simulink model "modeloexp10"  (R2015a)
settings: Solver=ode1  SolverMode=SingleTasking  StartTime=0.0  StopTime=10  FixedStep=0.01  RelTol=1e-3
values from neighbouring files (symbols this model uses):
  alfa = 0.2818    [exp10.m]
  K = 54.96    [exp10.m]
  Kc = 3    [exp10.m]
  KNL = 59.7881    [exp10.m]
  Kp = 1.604    [exp10.m]
  T = 0.27    [exp10.m]
  To = 0.134    [exp10.m]
  U = 1.59    [exp10.m]
undefined symbols (not defined in the file): phi
libraries: simulink x1
settings Model: CovExternalEMLEnable=on  Creator=rpm  LastModifiedBy=sasuk
settings DataIOCC: LimitDataPoints=off  SignalLoggingSaveFormat=ModelDataLogs  SaveOutput=off  SignalLogging=off  DSMLogging=off  SaveTime=off  TimeSaveName=t
settings OptimizationCC: ExpressionDepthLimit=2147483647  InitFltsAndDblsToZero=on
settings DebuggingCC: UnderspecifiedInitializationDetection=Classic  MergeDetectMultiDrivingBlocksExec=none  FcnCallInpInsideContextMsg=EnableAllAsWarning  StateNameClashWarn=warning
settings GRTTargetCC: CombineOutputUpdateFcns=off  GRTInterface=on

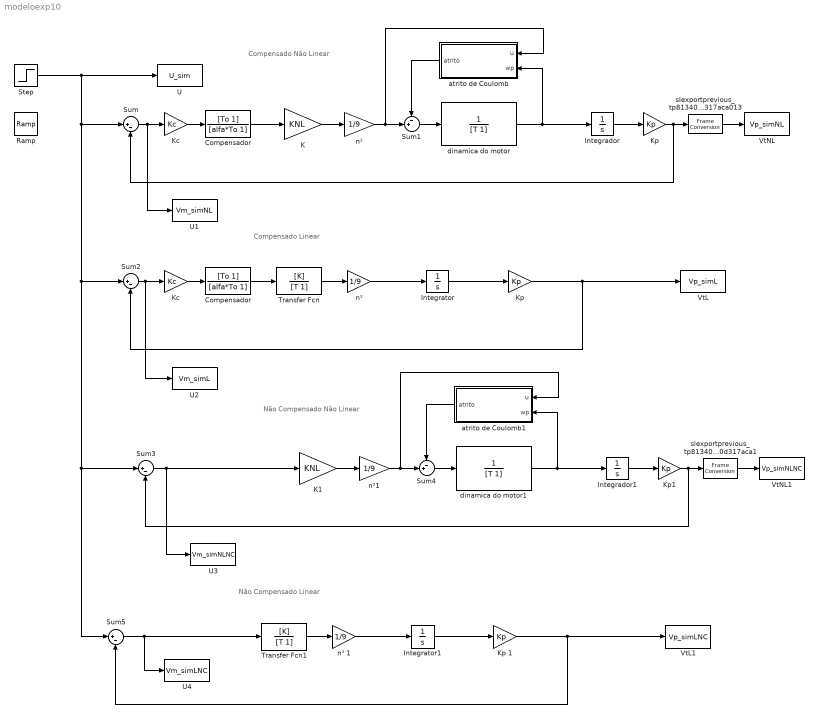
== system modeloexp10 ==
  note: Não Compensado
      | Não Linear
  note: Compensado Linear
  note: Compensado
      | Não
      | Linear
  note: Não Compensado Linear
  Compensador : TransferFcn  Numerator=[To 1]  Denominator=[alfa*To 1]
  "Compensador " : TransferFcn  Numerator=[To 1]  Denominator=[alfa*To 1]
  Integrador : Integrator
  Integrador1 : Integrator
  Integrator : Integrator
  Integrator1 : Integrator
  K : Gain  Gain=KNL
  K1 : Gain  Gain=KNL
  Kc : Gain  Gain=Kc
  "Kc " : Gain  Gain=Kc
  Kp : Gain  Gain=Kp
  "Kp " : Gain  Gain=Kp
  Kp 1 : Gain  Gain=Kp
  Kp1 : Gain  Gain=Kp
  Ramp : simulink/Sources/Ramp  slope=1  start=0  X0=0
  Step : Step  After=U  SampleTime=0
  Sum{,2..3,5} (4 alike) : Sum  Inputs=|+-
  Sum1 : Sum  Inputs=-+|
  Sum4 : Sum  Inputs=-+|
  Transfer Fcn : TransferFcn  Numerator=[K]  Denominator=[T 1]
  Transfer Fcn1 : TransferFcn  Numerator=[K]  Denominator=[T 1]
  U : ToWorkspace  VariableName=U_sim  SaveFormat=Timeseries  SampleTime=-1
  U1 : ToWorkspace  VariableName=Vm_simNL  SaveFormat=Timeseries  SampleTime=-1
  U2 : ToWorkspace  VariableName=Vm_simL  SaveFormat=Timeseries  SampleTime=-1
  U3 : ToWorkspace  VariableName=Vm_simNLNC  SaveFormat=Timeseries  SampleTime=-1
  U4 : ToWorkspace  VariableName=Vm_simLNC  SaveFormat=Timeseries  SampleTime=-1
  VtL : ToWorkspace  VariableName=Vp_simL  SaveFormat=Timeseries  SampleTime=-1
  VtL1 : ToWorkspace  VariableName=Vp_simLNC  SaveFormat=Timeseries  SampleTime=-1
  VtNL : ToWorkspace  VariableName=Vp_simNL  SaveFormat=Timeseries  SampleTime=-1
  VtNL1 : ToWorkspace  VariableName=Vp_simNLNC  SaveFormat=Timeseries  SampleTime=-1
  atrito de Coulomb : Subsystem  mask{phi=phi}
      mask Display: fprintf('phi = %3.1f', phi)
  atrito de Coulomb1 : Subsystem  mask{phi=phi}
      mask Display: fprintf('phi = %3.1f', phi)
  dinamica do motor : TransferFcn  Denominator=[T 1]
  dinamica do motor1 : TransferFcn  Denominator=[T 1]
  n² : Gain  Gain=1/9
  "n² " : Gain  Gain=1/9
  n² 1 : Gain  Gain=1/9
  n²1 : Gain  Gain=1/9
  slexportprevious_tp8134031d_9c58_445d_bef1_a0d317aca013 : FrameConversion  OutFrame=Sample-based
  slexportprevious_tp8134031d_9c58_445d_bef1_a0d317aca1 : FrameConversion  OutFrame=Sample-based
  wires:
  dinamica do motor/1 -> Integrador/1, atrito de Coulomb/2(wp)
  Integrador/1 -> Kp/1
  K/1 -> n²/1
  n²/1 -> atrito de Coulomb/1(u), Sum1/2
  atrito de Coulomb/1(atrito) -> Sum1/1
  Sum1/1 -> dinamica do motor/1
  Kp/1 -> Sum/2, slexportprevious_tp8134031d_9c58_445d_bef1_a0d317aca013/1
  slexportprevious_tp8134031d_9c58_445d_bef1_a0d317aca013/1 -> VtNL/1
  Transfer Fcn/1 -> "n² "/1
  "n² "/1 -> Integrator/1
  Integrator/1 -> "Kp "/1
  "Kp "/1 -> Sum2/2, VtL/1
  Sum/1 -> U1/1, Kc/1
  Kc/1 -> Compensador/1
  Compensador/1 -> K/1
  Sum2/1 -> U2/1, "Kc "/1
  "Kc "/1 -> "Compensador "/1
  "Compensador "/1 -> Transfer Fcn/1
  dinamica do motor1/1 -> Integrador1/1, atrito de Coulomb1/2(wp)
  Integrador1/1 -> Kp1/1
  K1/1 -> n²1/1
  n²1/1 -> atrito de Coulomb1/1(u), Sum4/2
  atrito de Coulomb1/1(atrito) -> Sum4/1
  Sum4/1 -> dinamica do motor1/1
  Kp1/1 -> Sum3/2, slexportprevious_tp8134031d_9c58_445d_bef1_a0d317aca1/1
  slexportprevious_tp8134031d_9c58_445d_bef1_a0d317aca1/1 -> VtNL1/1
  Sum3/1 -> U3/1, K1/1
  Transfer Fcn1/1 -> n² 1/1
  n² 1/1 -> Integrator1/1
  Integrator1/1 -> Kp 1/1
  Kp 1/1 -> Sum5/2, VtL1/1
  Sum5/1 -> U4/1, Transfer Fcn1/1
  Step/1 -> Sum5/1, Sum3/1, Sum2/1, Sum/1, U/1

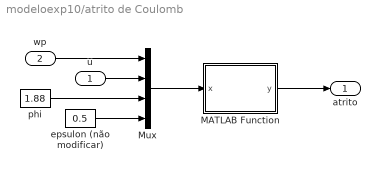
== system modeloexp10/atrito de Coulomb ==
  u : Inport
  wp : Inport  Port=2
  MATLAB Function : MATLAB Function  TreatAsAtomicUnit=on
  Mux : Mux
  epsulon (não modificar) : Constant  Value=0.5
  phi : Constant  Value=1.88
  atrito : Outport
  wires:
  u/1 -> Mux/2
  phi/1 -> Mux/3
  MATLAB Function/1(y) -> atrito/1
  wp/1 -> Mux/1
  epsulon (não modificar)/1 -> Mux/4
  Mux/1 -> MATLAB Function/1(x)

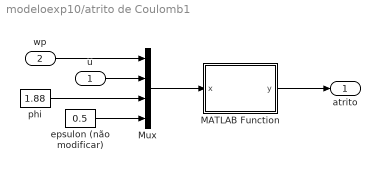
== system modeloexp10/atrito de Coulomb1 ==
  u : Inport
  wp : Inport  Port=2
  MATLAB Function : MATLAB Function  TreatAsAtomicUnit=on
  Mux : Mux
  epsulon (não modificar) : Constant  Value=0.5
  phi : Constant  Value=1.88
  atrito : Outport
  wires:
  u/1 -> Mux/2
  phi/1 -> Mux/3
  MATLAB Function/1(y) -> atrito/1
  wp/1 -> Mux/1
  epsulon (não modificar)/1 -> Mux/4
  Mux/1 -> MATLAB Function/1(x)

== matlab function modeloexp10/atrito de Coulomb1/MATLAB Function ==
  data: x input size=4; y output size=1
function y = nl_coulomb(x)
% Atrito de Coulomb
% Para uso de nl_template.mdl

wp  = x(1); 
u   = x(2); 
phi = x(3); 
epsulon = x(4);

y = 0;

if wp > epsulon
    y = phi;
elseif wp < -epsulon
    y = -phi;
elseif wp >= 0
    y = min(phi,abs(u));
elseif wp < 0
    y = max(-phi,-abs(u));
end

== matlab function modeloexp10/atrito de Coulomb/MATLAB Function ==
  data: x input size=4; y output size=1
function y = nl_coulomb(x)
% Atrito de Coulomb
% Para uso de nl_template.mdl

wp  = x(1); 
u   = x(2); 
phi = x(3); 
epsulon = x(4);

y = 0;

if wp > epsulon
    y = phi;
elseif wp < -epsulon
    y = -phi;
elseif wp >= 0
    y = min(phi,abs(u));
elseif wp < 0
    y = max(-phi,-abs(u));
end
